simulink model "flatsat_data_send"  (R2021a)
settings: Solver=VariableStepAuto  StartTime=0.0  StopTime=Inf  RelTol=1e-3
values from neighbouring files (symbols this model uses):
  t_send = 1/25    (= 0.04)    [flatsat_data_send_init.m]
undefined symbols (not defined in the file or in its folder): t_recieve
libraries: instrumentseriallib x3
settings Model: EnablePacing=on  Creator=Alex Zhen  LastModifiedBy=Alex Zhen
settings SolverCC: AlgebraicLoopSolver=TrustRegion
settings DebuggingCC: SFMachineParentedDataDiag=warning  ArithmeticOperatorsInVariantConditions=warning
settings SFSimCC: CustomCodeUndefinedFunction=UseInterfaceOnly

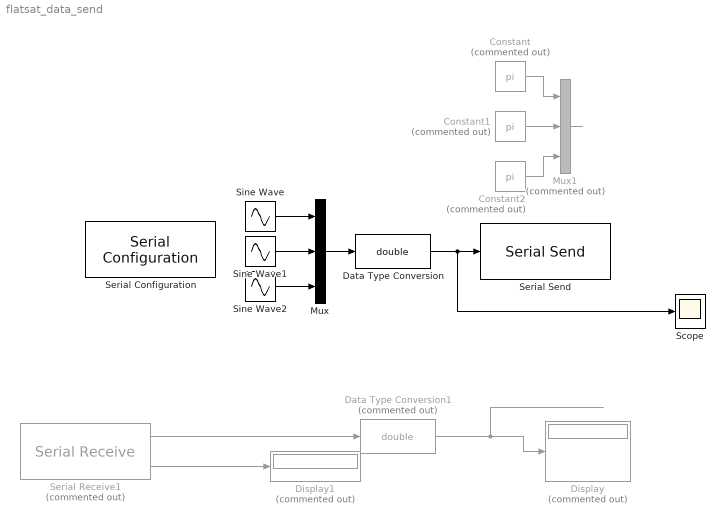
== system flatsat_data_send ==
  Constant : Constant  Commented=on  Value=pi  SampleTime=t_send
  Constant1 : Constant  Commented=on  Value=pi  SampleTime=t_send
  Constant2 : Constant  Commented=on  Value=pi  SampleTime=t_send
  Data Type Conversion : DataTypeConversion  OutDataTypeStr=double
  Data Type Conversion1 : DataTypeConversion  Commented=on  OutDataTypeStr=double
  Display : Display  Commented=on
  Display1 : Display  Commented=on
  Mux : Mux  Inputs=3
  Mux1 : Mux  Commented=on  Inputs=3
  Scope : Scope
  Serial Configuration : instrumentseriallib/Serial Configuration  Priority=-200000  Port=COM9  ComPort=COM9  BaudRate=115200  DataBits=8  Parity=none  StopBits=1  ByteOrder=little-endian  FlowControl=none  Timeout=10  SimulateUsing=Interpreted execution  BlockInModel=on
  Serial Receive1 : instrumentseriallib/Serial Receive  Commented=on  Port=<Select a port...>  ComPort=<Please select a port...>  DataType=double  SaveDataType=uint8  ToggleHeader=off  Header=[]  ToggleTerminator=on  Terminator=<none>  CustomTerminator=[]  ToggleDataSize=on  DataSize="[3  1]"  EnableBlockingMode=off  ActionDataUnavailable=Output last received value  ActionWhenDataUnavailable=Output last received value  CustomValue=0  SampleTime=t_recieve  SimulateUsing=Interpreted execution  BlockInModel=on
  Serial Send : instrumentseriallib/Serial Send  Port=COM9  ComPort=COM9  Header=[]  Terminator=<none>  CustomTerminator=[]  EnableBlockingMode=off  SimulateUsing=Interpreted execution  BlockInModel=on
  Sine Wave : Sin  Amplitude=250  Frequency=pi/5  SampleTime=t_send
  Sine Wave1 : Sin  Amplitude=250  Frequency=pi/5  Phase=1  SampleTime=t_send
  Sine Wave2 : Sin  Amplitude=250  Frequency=pi/5  Phase=2  SampleTime=t_send
  wires:
  Sine Wave/1 -> Mux/1
  Serial Receive1/1 -> Data Type Conversion1/1
  Data Type Conversion/1 -> Scope/1, Serial Send/1
  Serial Receive1/2 -> Display1/1
  Data Type Conversion1/1 -> Display/1
  Sine Wave1/1 -> Mux/2
  Sine Wave2/1 -> Mux/3
  Mux/1 -> Data Type Conversion/1
  Constant1/1 -> Mux1/2
  Constant/1 -> Mux1/1
  Constant2/1 -> Mux1/3
  Mux1/1 -> ?
